simulink model "rrScenarioSimWithSensors"  (R2024b)
settings: Solver=FixedStepAuto  StartTime=0  StopTime=10  FixedStep=simStepSize  RelTol=1e-3
values from neighbouring files (symbols this model uses):
  simStepSize = 0.1    [RunThis.m]    (also in TestTest.m)
undefined symbols (not defined in the file or in its folder): Defined, driving, Ego, Lane, User
libraries: roadrunnerscenario x7, drivingscenarioandsensors x1
settings Model: Creator=The MathWorks, Inc.  LastModifiedBy=andre
settings DataIOCC: LimitDataPoints=on  MaxDataPoints=100  SaveFormat=StructureWithTime  SaveOutput=off  DSMLogging=off  DatasetSignalFormat=timetable
settings OptimizationCC: ReuseModelBlockBuffer=off
settings DebuggingCC: SubsystemReferenceDiagnosticForUnitTest=warning
settings RTWCC: GPUComputeCapability=3.5

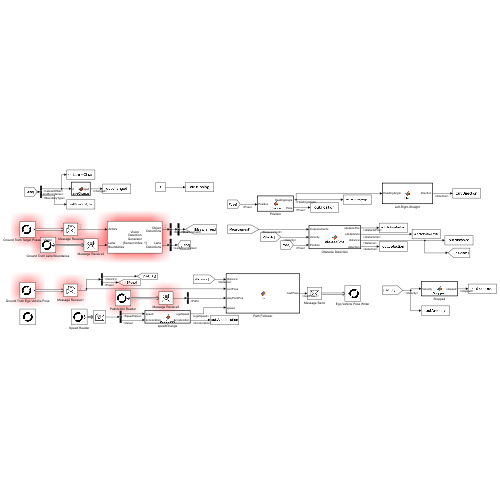
[thumbnail: Simulink's stored preview of the top-level diagram]
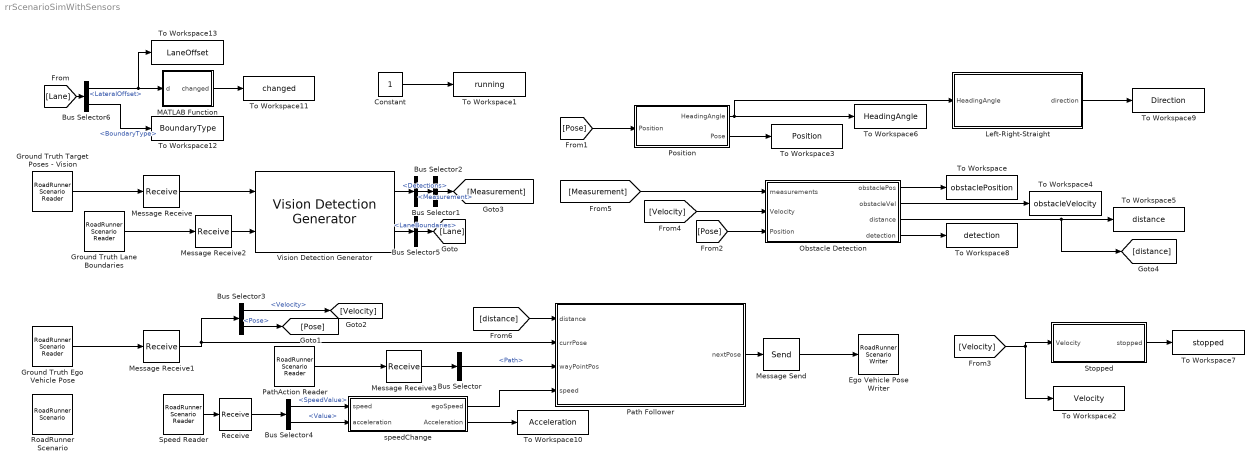
== system rrScenarioSimWithSensors ==
  Bus Selector : BusSelector  OutputSignals=PathTarget.Path
  Bus Selector1 : BusSelector  OutputSignals=Measurement
  Bus Selector2 : BusSelector  OutputSignals=Detections
  Bus Selector3 : BusSelector  OutputSignals=Velocity,Pose
  Bus Selector4 : BusSelector  OutputSignals=SpeedTarget.SpeedValue,TransitionDynamics.Value
  Bus Selector5 : BusSelector  OutputSignals=LaneBoundaries
  Bus Selector6 : BusSelector  OutputSignals=LateralOffset,BoundaryType
  Constant : Constant
  Ego Vehicle Pose Writer : roadrunnerscenario/RoadRunner Scenario Writer  TopicCategory=Actor  ActorCategory=All Types  EventType=Action Complete  UserDefinedEvent=Event1  VehicleType=Vehicle Pose  TopicType=Actor Pose
  Ground Truth Ego Vehicle Pose : roadrunnerscenario/RoadRunner Scenario Reader  TopicCategory=Actor  ActorCategory=All Types  ActionType=Path Following  EventType=User-Defined  TopicType=Actor Pose  VehicleType=Vehicle Pose  UserDefinedAction=Action1  UserDefinedEvent=Event1  Filter=Self  SensorTopic=Target Poses  LaneBoundaryOutputTopic=Ego-Lane  SensorID=1  SampleTime=simStepSize
  Ground Truth Lane Boundaries : roadrunnerscenario/RoadRunner Scenario Reader  TopicCategory=Sensor  ActorCategory=All Types  ActionType=Path Following  EventType=User-Defined  TopicType=Actor Pose  VehicleType=Vehicle Pose  UserDefinedAction=Action1  UserDefinedEvent=Event1  Filter=Self  SensorTopic=Lane Boundaries  LaneBoundaryOutputTopic=Ego and Adjacent Lanes  SensorID=1  SampleTime=simStepSize
  Ground Truth Target Poses - Vision : roadrunnerscenario/RoadRunner Scenario Reader  TopicCategory=Sensor  ActorCategory=All Types  ActionType=Path Following  EventType=User-Defined  TopicType=Actor Specifications  VehicleType=Vehicle Specifications  UserDefinedAction=Action1  UserDefinedEvent=Event1  Filter=Self  SensorTopic=Target Poses  LaneBoundaryOutputTopic=Ego-Lane  SensorID=1  SampleTime=simStepSize
  Left-Right-Straight : MATLAB Function  TreatAsAtomicUnit=on
  MATLAB Function : MATLAB Function  TreatAsAtomicUnit=on
  Message Receive{,1..3} (4 alike) : Receive  InputPortMessageModes=m  UseInternalQueue=off  SampleTime=simStepSize
  Message Send : Send  OutputPortMessageModes=m
  Obstacle Detection : MATLAB Function  TreatAsAtomicUnit=on
  Path Follower : MATLAB Function  TreatAsAtomicUnit=on
  PathAction Reader : roadrunnerscenario/RoadRunner Scenario Reader  TopicCategory=Action  ActorCategory=All Types  ActionType=Path Following  EventType=User-Defined  TopicType=Actor Specifications  VehicleType=Vehicle Specifications  UserDefinedAction=Action1  UserDefinedEvent=Event1  Filter=Self  SensorTopic=Target Poses  LaneBoundaryOutputTopic=Ego-Lane  SensorID=1  SampleTime=simStepSize
  Position : MATLAB Function  TreatAsAtomicUnit=on
  Receive : Receive  InputPortMessageModes=m  UseInternalQueue=off  QueueOverwriting=on  QueueLength=1  QueueType=LIFO
  RoadRunner Scenario : roadrunnerscenario/RoadRunner Scenario  UserDefinedActions={}  UserDefinedEvents={}
  Speed Reader : roadrunnerscenario/RoadRunner Scenario Reader  TopicCategory=Action  ActorCategory=All Types  ActionType=Speed Change  EventType=User-Defined  TopicType=Actor Specifications  VehicleType=Vehicle Specifications  UserDefinedAction=Action1  UserDefinedEvent=Event1  Filter=Self  SensorTopic=Target Poses  LaneBoundaryOutputTopic=Ego-Lane  SensorID=1  SampleTime=0
  Stopped : MATLAB Function  TreatAsAtomicUnit=on
  To Workspace : ToWorkspace  VariableName=obstaclePosition  SaveFormat=Timeseries  SampleTime=-1
  To Workspace1 : ToWorkspace  VariableName=running  SaveFormat=Timeseries  SampleTime=-1
  To Workspace10 : ToWorkspace  VariableName=Acceleration  SaveFormat=Timeseries  SampleTime=-1
  To Workspace11 : ToWorkspace  VariableName=changed  SaveFormat=Timeseries  SampleTime=-1
  To Workspace12 : ToWorkspace  VariableName=BoundaryType  SaveFormat=Timeseries  SampleTime=-1
  To Workspace13 : ToWorkspace  VariableName=LaneOffset  SaveFormat=Timeseries  SampleTime=-1
  To Workspace2 : ToWorkspace  VariableName=Velocity  SaveFormat=Timeseries  SampleTime=-1
  To Workspace3 : ToWorkspace  VariableName=Position  SaveFormat=Timeseries  SampleTime=-1
  To Workspace4 : ToWorkspace  VariableName=obstacleVelocity  SaveFormat=Timeseries  SampleTime=-1
  To Workspace5 : ToWorkspace  VariableName=distance  SaveFormat=Timeseries  SampleTime=-1
  To Workspace6 : ToWorkspace  VariableName=HeadingAngle  SaveFormat=Timeseries  SampleTime=-1
  To Workspace7 : ToWorkspace  VariableName=stopped  SaveFormat=Timeseries  SampleTime=-1
  To Workspace8 : ToWorkspace  VariableName=detection  SaveFormat=Timeseries  SampleTime=-1
  To Workspace9 : ToWorkspace  VariableName=Direction  SaveFormat=Timeseries  SampleTime=-1
  Vision Detection Generator : drivingscenarioandsensors/Vision Detection Generator  SensorIndex=1  DetectorOutput=Lanes and objects  UpdateInterval=simStepSize  LaneUpdateInterval=simStepSize  SensorLocation=[1.2 0]  Height=1.1  Yaw=0  Pitch=1  Roll=0  BusNameSource=Auto  BusName=BusObjectDetections  BusName2Source=Auto  BusName2=BusLaneDetections  MaxNumDetectionsSource=Property  MaxNumDetections=1  MaxNumLanesSource=Property  MaxNumLanes=1  DetectionCoordinates=Ego Cartesian  SimulateUsing=Interpreted execution  MaxRange=150  BoundingBoxAccuracy=5  ProcessNoiseIntensity=5  MaxSpeed=100  MaxAllowedOcclusion=0.5  MinObjectImageSize=[ 15, 15 ]  DetectionProbability=1  FalsePositivesPerImage=0  MinLaneImageSize=[ 20, 3 ]  LaneBoundaryAccuracy=3  HasNoise=off  InitialSeedSource=Repeatable  InitialSeed=0  UsedSeed=driving.internal.SimulinkUtilities.seedManager(gcb)  ActorProfilesSource=From Scenario Reader block  ActorProfilesParameters=driving.internal.ActorProfilesParameters  ActorProfilesExpression=actorProfiles  Intrinsics=driving.internal.cameraIntrinsics('FocalLength',[ 1200, 1200 ])
  speedChange : MATLAB Function  TreatAsAtomicUnit=on
  wires:
  Ground Truth Target Poses - Vision/1 -> Message Receive/1
  Ground Truth Ego Vehicle Pose/1 -> Message Receive1/1
  Path Follower/1(nextPose) -> Message Send/1
  PathAction Reader/1 -> Message Receive3/1
  Message Receive3/1 -> Bus Selector/1
  Message Send/1 -> Ego Vehicle Pose Writer/1
  Bus Selector/1 -> Path Follower/3(wayPointPos)  "<Path>"
  Ground Truth Lane Boundaries/1 -> Message Receive2/1
  Bus Selector2/1 -> Bus Selector1/1  "<Detections>"
  Message Receive1/1 -> Bus Selector3/1, Path Follower/2(currPose)
  Bus Selector3/1 -> [Velocity]  "<Velocity>"
  Bus Selector3/2 -> [Pose]  "<Pose>"
  Constant/1 -> To Workspace1/1
  Message Receive2/1 -> Vision Detection Generator/2
  Message Receive/1 -> Vision Detection Generator/1
  Speed Reader/1 -> Receive/1
  Receive/1 -> Bus Selector4/1
  Bus Selector4/2 -> speedChange/2(acceleration)  "<Value>"
  Bus Selector4/1 -> speedChange/1(speed)  "<SpeedValue>"
  speedChange/1(egoSpeed) -> Path Follower/4(speed)
  Bus Selector1/1 -> [Measurement]  "<Measurement>"
  Obstacle Detection/1(obstaclePos) -> To Workspace/1
  Obstacle Detection/3(distance) -> [distance], To Workspace5/1
  Obstacle Detection/2(obstacleVel) -> To Workspace4/1
  Position/2(Pose) -> To Workspace3/1
  Stopped/1(stopped) -> To Workspace7/1
  Obstacle Detection/4(detection) -> To Workspace8/1
  Position/1(HeadingAngle) -> To Workspace6/1, Left-Right-Straight/1(HeadingAngle)
  Left-Right-Straight/1(direction) -> To Workspace9/1
  speedChange/2(Acceleration) -> To Workspace10/1
  Vision Detection Generator/2 -> Bus Selector5/1
  Bus Selector6/1 -> MATLAB Function/1(d), To Workspace13/1  "<LateralOffset>"
  MATLAB Function/1(changed) -> To Workspace11/1
  [Lane] -> Bus Selector6/1
  Bus Selector5/1 -> [Lane]  "<LaneBoundaries>"
  [Pose] -> Position/1(Position)
  [Pose] -> Obstacle Detection/3(Position)
  [Velocity] -> To Workspace2/1, Stopped/1(Velocity)
  [Velocity] -> Obstacle Detection/2(Velocity)
  [Measurement] -> Obstacle Detection/1(measurements)
  [distance] -> Path Follower/1(distance)
  Vision Detection Generator/1 -> Bus Selector2/1
  Bus Selector6/2 -> To Workspace12/1  "<BoundaryType>"

== matlab function rrScenarioSimWithSensors/speedChange ==
  data: speed input; egoSpeed output; acceleration input; simStepSize parameter; Acceleration output
function [egoSpeed, Acceleration]= egoSpeed(speed,acceleration,simStepSize)

persistent currSpeed

%Initializes first speed value
if isempty(currSpeed)
    currSpeed=speed;
end

%Sets egoSpeed to current Speed
egoSpeed=currSpeed;

%Tests to see if the car is accelerating or deccelerating
sign=1;
if currSpeed>speed
    sign=-1;
end

%Outputs Acceleration Values for Potential Test
Acceleration=sign*acceleration;

%Calculates change in speed from acceleration value and simulation step
%time
speedChange=sign*acceleration*simStepSize;

%Ensures speed value is not overshot
if abs(currSpeed-speed)>speedChange
    currSpeed=currSpeed+speedChange;
else
    currSpeed=speed;
end

end

== matlab function rrScenarioSimWithSensors/Path Follower ==
  data: distance input; currPose input; wayPointPos input; nextPose output Bus: BusActorRuntime; simStepSize parameter; speed input
function nextPose  = fcn(distance, currPose, wayPointPos,simStepSize,speed)
%Updates current Speed
egoSpeed  = speed;

%Strips unnecessary waypoints 
persistent wPP
if isempty(wPP)
    wPP = reshape(wayPointPos(wayPointPos~=0),[],2);
end

%Index 1 is the closest waypoint
nWPP=wPP(1,:);

%Sets current point goal
currPoint = [currPose.Pose(1,4) currPose.Pose(2,4)];

%Distance between current point and next way point
delXY = nWPP-currPoint;

%Distance between current point and next way point
dist = norm(delXY);

%Runs through points until the next point is over the distance travelled by
%the car
while dist<(egoSpeed*simStepSize)
    wPP(1,:)=[];
    nWPP=wPP(1,:);
    delXY = nWPP-currPoint;
    dist = norm(delXY);
end 

%Sets heading angle between points
hAngle = atan2d(delXY(2),delXY(1));

%Writes new points for the car to go to
nextPose = currPose;

%New Point Position (x and y values)
nextPose.Pose(1,4) = nextPose.Pose(1,4)+egoSpeed*simStepSize*cosd(hAngle);
nextPose.Pose(2,4) = nextPose.Pose(2,4)+egoSpeed*simStepSize*sind(hAngle);

%Heading Angle Values
nextPose.Pose(1:3,1:3) = [cosd(hAngle-90) -sind(hAngle-90) 0;...
                          sind(hAngle-90) cosd(hAngle-90) 0;...
                          0 0 1];

%Updates Car Velocity
nextPose.Velocity=[egoSpeed*cosd(hAngle) egoSpeed*sind(hAngle) 0];
end

== matlab function rrScenarioSimWithSensors/Obstacle Detection ==
  data: measurements input; Velocity input; Position input; obstaclePos output; obstacleVel output; distance output; detection output
function [obstaclePos,obstacleVel,distance,detection] = obstacleData(measurements, Velocity, Position)
    %Assumes car is being detected
    detection=true;

    %Relative Position and Velocity
    relPos=[measurements(1) measurements(2) measurements(3)];
    relVel=[measurements(4) measurements(5) measurements(6)];

    %Distance between Autonomous Vehicle and Detected Car
    distance=norm(relPos);

    %Transformation Matrix for adjusting relative Position to absolute
    %Position
    tMat=[Position(1,1) Position(1,2) 0;...
          Position(2,1) Position(2,2) 0;
          0 0 1];

    %Checks if car is actually being detected
    if relPos==[0 0 0]
        detection=false;
    end

    %Sets absolute position and velocities of detected cars
    absRelPos=relPos*tMat;
    obstaclePos=absRelPos+[Position(1,4) Position(2,4) Position(3,4)];
    absRelVel=relVel*tMat;
    obstacleVel=absRelVel+Velocity;
end

== matlab function rrScenarioSimWithSensors/Position ==
  data: HeadingAngle output; Position input; Pose output
function [HeadingAngle,Pose] = position(Position)
    %Reformats bus value to have position in cartesian coordinates and
    %heading angle in degrees
    Pose=[Position(1,4) Position(2,4) Position(3,4)];
    HeadingAngle=atan2d(Position(2,1),Position(1,1));
end

== matlab function rrScenarioSimWithSensors/Left-Right-Straight ==
  data: HeadingAngle input; direction output
%Determines the Heading Angle of Autonomous Vehicle
function direction = LRS(HeadingAngle)
    persistent hA
    %Sets initial Heading Angle
    if isempty(hA)
        hA=HeadingAngle;
    end
    
    %Calculates the difference between current angle and previous angle
    lrs=int16(1000*(hA-HeadingAngle));

    %Determines if car turns left or right based on change in angle
    if lrs<0
        direction="Left";
    elseif lrs>0
        direction="Right";
    else
        direction="Straight";
    end
    hA=HeadingAngle;
end

== matlab function rrScenarioSimWithSensors/Stopped ==
  data: Velocity input; stopped output
%Checks if a car is stopped
function stopped = Stopped(Velocity)
    %Car is assumed to be in motion
    stopped=false;
    
    %If velocity is 0 in all axes, it is stopped
    if norm(Velocity)==0
        stopped=true;
    end
end

== matlab function rrScenarioSimWithSensors/MATLAB Function ==
  data: changed output; d input
function changed = laneChange(d)
    persistent dist
    if isempty(dist)
       dist=d;
    end
    if isnan(dist)
        dist=d;
    end
    if ~isnan(d)
        if dist*d>=0
            changed=false;
        else 
            changed=true;
        end
    else
        changed=false;
    end
    dist=d;
end
